simulink model "system_mdl"  (R2021a)
settings: Solver=FixedStepAuto  StartTime=0  StopTime=1  FixedStep=0.0001  RelTol=1e-3
values from neighbouring files (symbols this model uses):
  A = [0 1 0 ... (first row only)    [valueIteration.m]
  B = [0 0 1/T_d0]'    [valueIteration.m]
  K = p(n*n+1:n*n+n*m)'    [valueIteration.m]
  T_smpl_sim = 0.0001    [valueIteration.m]
  x0 = x(end,:)'+x_eq    [valueIteration.m]
  x_eq = [delta_0 0 P_m0]'    [valueIteration.m]
settings Model: Creator=Hamad  LastModifiedBy=Hamad

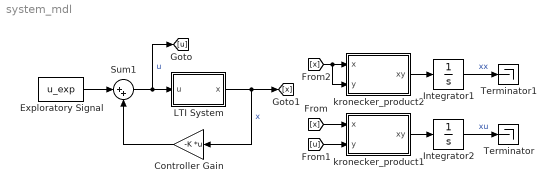
== system system_mdl ==
  Controller Gain : Gain  Gain=-K  Multiplication=Matrix(K*u)
  Exploratory Signal : FromWorkspace  VariableName=u_exp  SampleTime=T_smpl_sim  OutputAfterFinalValue=Setting to zero
  Integrator1 : Integrator
  Integrator2 : Integrator
  LTI System : Subsystem
  Sum1 : Sum  Inputs=|++
  Terminator : Terminator
  Terminator1 : Terminator
  kronecker_product1 : MATLAB Function  TreatAsAtomicUnit=on
  kronecker_product2 : MATLAB Function  TreatAsAtomicUnit=on
  wires:
  Integrator1/1 -> Terminator1/1  "xx"
  kronecker_product1/1(xy) -> Integrator2/1
  Integrator2/1 -> Terminator/1  "xu"
  Controller Gain/1 -> Sum1/2
  Exploratory Signal/1 -> Sum1/1
  Sum1/1 -> [u], LTI System/1(u)  "u"
  kronecker_product2/1(xy) -> Integrator1/1
  [u] -> kronecker_product1/2(y)
  [x] -> kronecker_product1/1(x)
  [x] -> kronecker_product2/2(y), kronecker_product2/1(x)
  LTI System/1(x) -> [x], Controller Gain/1  "x"

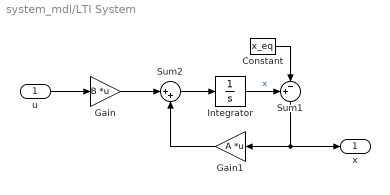
== system system_mdl/LTI System ==
  u : Inport
  Constant : Constant  Value=x_eq
  Gain : Gain  Gain=B  Multiplication=Matrix(K*u)
  Gain1 : Gain  Gain=A  Multiplication=Matrix(K*u)
  Integrator : Integrator  InitialCondition=x0
  Sum1 : Sum  Inputs=+-|
  Sum2 : Sum  Inputs=|++
  x : Outport
  wires:
  Sum2/1 -> Integrator/1
  Integrator/1 -> Sum1/1  "x"
  Gain/1 -> Sum2/1
  u/1 -> Gain/1
  Gain1/1 -> Sum2/2
  Constant/1 -> Sum1/2
  Sum1/1 -> x/1, Gain1/1

== matlab function system_mdl/kronecker_product1 ==
  data: x input; xy output; y input
function xy = kron(x,y)

temp = x*y';
xy = temp(:);
end

== matlab function system_mdl/kronecker_product2 ==
  data: x input; xy output; y input
function xy = kron(x,y)

temp = x*y';
xy = temp(:);
end
